simulink model "three_dof_simulink"  (R2024b)
settings: Solver=VariableStepAuto  StartTime=0.0  StopTime=200  RelTol=1e-3
undefined symbols (not defined in the file or in its folder): aeroList, pfoilList
libraries: aerolibanim x1, simulink x1
settings Model: Creator=bgbg0  LastModifiedBy=bgbg0

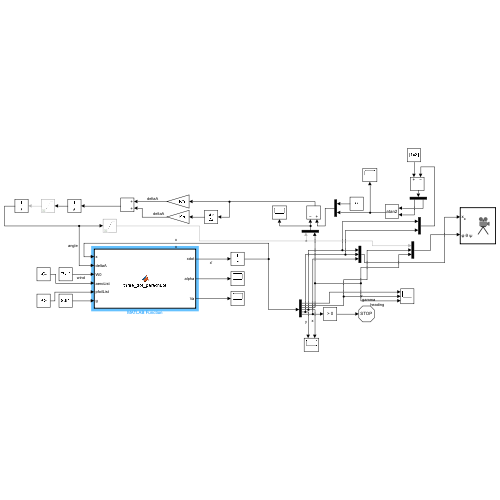
[thumbnail: Simulink's stored preview of the top-level diagram]
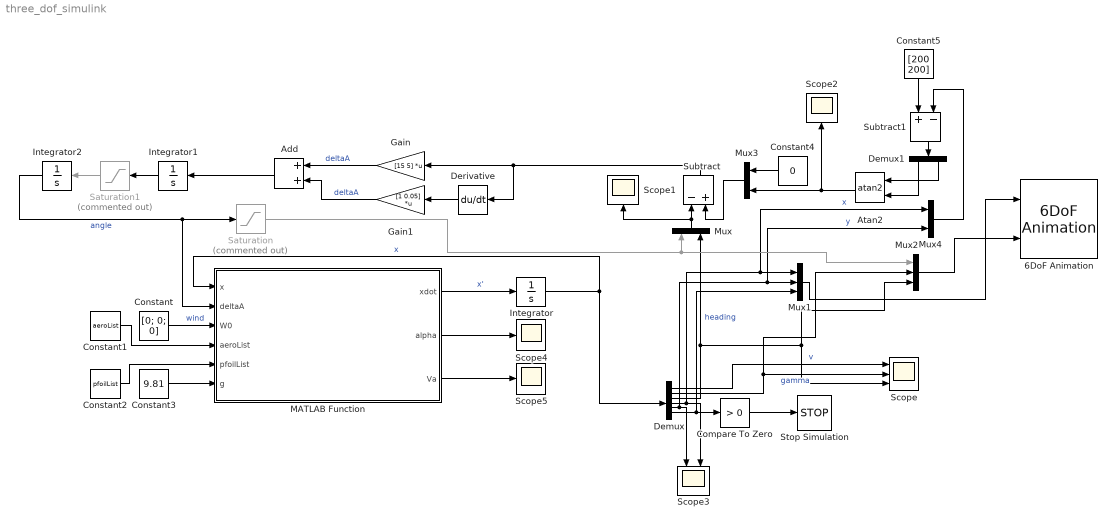
== system three_dof_simulink ==
  6DoF Animation : aerolibanim/6DoF Animation  u1=[-100 100 -100 100 -200 0]  u2=0.1  u3=1.0  u4=[0 0 0]  u5=Fly alongside  u6=[2000 500 -3150]  u7=10  u8=on
  Add : Sum
  Atan2 : Trigonometry  Operator=atan2
  Compare To Zero : simulink/Logic and Bit Operations/Compare To Zero  relop=>  OutDataTypeStr=boolean
  Constant : Constant  Value=[0; 0; 0]
  Constant1 : Constant  Value=aeroList
  Constant2 : Constant  Value=pfoilList
  Constant3 : Constant  Value=9.81
  Constant4 : Constant  Value=0
  Constant5 : Constant  Value=[200 200]
  Demux : Demux  Outputs=6
  Demux1 : Demux  Outputs=2
  Derivative : Derivative
  Gain : Gain  Gain=[15 5]  Multiplication=Matrix(K*u)
  Gain1 : Gain  Gain=[1 0.05]  Multiplication=Matrix(K*u)
  Integrator : Integrator  InitialCondition=[10 0 0 0 0 -500]
  Integrator1 : Integrator
  Integrator2 : Integrator
  MATLAB Function : MATLAB Function  TreatAsAtomicUnit=on
  Mux : Mux  Inputs=2
  Mux1 : Mux  Inputs=3
  Mux2 : Mux  Inputs=3
  Mux3 : Mux  Inputs=2
  Mux4 : Mux  Inputs=2
  Saturation : Saturate  Commented=on
  Saturation1 : Saturate  Commented=on
  Scope : Scope  NumInputPorts=3
  Scope{1..2,4..5} (4 alike) : Scope
  Scope3 : Scope  NumInputPorts=2
  Stop Simulation : Stop
  Subtract : Sum  Inputs=-+
  Subtract1 : Sum  Inputs=+-
  wires:
  MATLAB Function/1(xdot) -> Integrator/1  "x'"
  Integrator/1 -> Demux/1, MATLAB Function/1(x)  "x"
  Constant3/1 -> MATLAB Function/6(g)
  Gain/1 -> Add/1  "deltaA"
  Constant/1 -> MATLAB Function/3(W0)  "wind"
  Constant1/1 -> MATLAB Function/4(aeroList)
  Constant2/1 -> MATLAB Function/5(pfoilList)
  Demux/6 -> Mux1/3, Compare To Zero/1
  Compare To Zero/1 -> Stop Simulation/1
  Subtract/1 -> Derivative/1, Gain/1
  Constant4/1 -> Mux3/1
  Demux/3 -> Mux2/3, Scope/3, Mux/2  "heading"
  Mux/1 -> Scope1/1, Subtract/1
  Integrator1/1 -> Saturation1/1
  Integrator2/1 -> MATLAB Function/2(deltaA), Saturation/1  "angle"
  Demux/1 -> Scope/1  "v"
  Demux/2 -> Mux2/2, Scope/2  "gamma"
  Demux/4 -> Scope3/2, Mux4/1, Mux1/1  "x"
  Demux/5 -> Scope3/1, Mux4/2, Mux1/2  "y"
  Mux1/1 -> 6DoF Animation/1
  Mux2/1 -> 6DoF Animation/2
  Derivative/1 -> Gain1/1
  Gain1/1 -> Add/2  "deltaA"
  Mux3/1 -> Subtract/2
  Atan2/1 -> Scope2/1, Mux3/2
  Mux4/1 -> Subtract1/2
  Constant5/1 -> Subtract1/1
  Subtract1/1 -> Demux1/1
  Demux1/1 -> Atan2/2
  Demux1/2 -> Atan2/1
  Add/1 -> Integrator1/1
  Saturation/1 -> Mux/1, Mux2/1
  Saturation1/1 -> Integrator2/1
  MATLAB Function/2(alpha) -> Scope4/1
  MATLAB Function/3(Va) -> Scope5/1

== matlab function three_dof_simulink/MATLAB Function ==
  data: x input; xdot output; deltaA input; W0 input; aeroList input; pfoilList input; g input; alpha output; Va output
% 3 DOF from DARTS 
% started 06/10/24 - Rosalind Aves

function [xdot, alpha, Va] = three_dof_parachute(x, deltaA, W0, aeroList, pfoilList, g)

cell = num2cell(pfoilList);
[pfoilParams.b, pfoilParams.c, pfoilParams.S, pfoilParams.AR, pfoilParams.t, pfoilParams.mu, pfoilParams.eps, pfoilParams.a, pfoilParams.R, pfoilParams.d, pfoilParams.n, pfoilParams.m_s, pfoilParams.m_p, pfoilParams.A_cube, pfoilParams.l_cont] = cell{:};
Va_norm = x(1);
gamma = x(2);
Psi = x(3); % heading angle
X = x(4);
Y = x(5);
Z = x(6);

% if (abs(Z) < 2825) % pretied
%     deltaA = -delta(2);
% else
%     deltaA = 0;
% end

% if (abs(Z) < 2491) && (abs(Z) > 2357) % 50 sec actuation
%     deltaA = delta(2);
% elseif (abs(Z) < 2357) && (abs(Z) > 2241) % 20 sec hold neutral
%     deltaA = 0;
% elseif (abs(Z) < 2241) % rest of flight actuation
%     deltaA = -delta(2);
% else
%     deltaA = 0;
% end

S = pfoilParams.S;
m = pfoilParams.m_s;
rho = 1.225; % atmos(Z, 4);
phi = deltaA; % bank angle (set to 0 if no control)
W = W0; % wind vector - inertial

R_WN = [cos(Psi)*cos(gamma) sin(Psi)*cos(gamma) -sin(gamma); ...
        cos(Psi)*sin(gamma)*sin(phi) - sin(Psi)*cos(phi) sin(Psi)*sin(gamma)*sin(phi) + cos(Psi)*cos(phi) cos(gamma)*sin(phi); ...
        cos(Psi)*sin(gamma)*cos(phi) + sin(Psi)*sin(phi) sin(Psi)*sin(gamma)*cos(phi) - cos(Psi)*sin(phi) cos(gamma)*cos(phi)];

V = R_WN' * [Va_norm; 0; 0] + R_WN * W;
Va = V - R_WN * W;
alpha = atan(abs(Va(3) / sqrt(Va(1)^2 + Va(2)^2)));


% Aerodynamic and control coefficients
CL_0 = aeroList(3);
CL_alpha= 0.9; %aeroParams.CLalpha;
CL_deltas = aeroList(28);

CD_0= aeroList(5);
CD_s = aeroList(6);
CD_l = (pfoilParams.n .* pfoilParams.R .* pfoilParams.d .* cos(alpha).^3) ./ S;
CD_deltas = ((CL_alpha^2/(aeroList(2)*pfoilParams.AR*pi)) * (alpha - aeroList(1) - aeroList(25))^2 + aeroList(27)) * 2 * aeroList(23);

CL = CL_0 + CL_alpha * alpha + CL_deltas * (abs(deltaA)); %lift coefficient
CD = CD_0 + CD_s + CD_l + CL_alpha.^2 .* (alpha*cos(pfoilParams.eps/2) - aeroList(1)).^2 / (aeroList(2)*pfoilParams.AR*pi) + CD_deltas*(abs(deltaA));

% if alpha < -0.5 || alpha > 0.5
%     CL = 0;
%     CD = 1;
% end

% Lift and Drag
% CL = 0.2985;
% CD = CL;
L = 0.5 * rho * Va_norm^2 * S * CL;
D = 0.5 * rho * Va_norm^2 * S * CD;

% A = [sin(gamma)*Va -cos(gamma)*cos(phi)*Va; (m*cos(gamma)*Va) (m*cos(gamma)*sin(phi)*Va)];
% b = [-g*cos(gamma)*sin(gamma); (L-m*g*cos(gamma)*cos(phi))];

% omegaDOT = A\b;
xdot = zeros(1, 6);
xdot(1) = -1/m * (D + m*g*sin(gamma));
xdot(2) = 1/(m*Va_norm) * (L*cos(phi) - m*g*cos(gamma));
xdot(3) = (L*sin(phi)) / (m*Va_norm*cos(gamma));
xdot(4:6) = R_WN' * [Va_norm; 0; 0] + W;
end
